simulink model "s_sip_lqr"  (Simulink 7.8)
settings: Solver=ode4  StartTime=0.0  StopTime=10  FixedStep=0.002  RelTol=1e-3  AbsTol=1e-6
values from neighbouring files (symbols this model uses):
  A = [0 0 1 0 ... (first row only)    [SIP_ABCD_eqns.m]
  B = eta_g*Kg*eta_m*Kt/r_mp/Rm*B    [SIP_ABCD_eqns.m]
  C = eye(2,4)    [SIP_ABCD_eqns.m]    (also in d_ip02_sip_lqr.m = eye( 4 ))
  D = zeros(2,1)    [SIP_ABCD_eqns.m]    (also in d_ip02_sip_lqr.m = zeros( 4, 1 ))
  IC_ALPHA0 = IC_ALPHA0 / 180 * pi    (= 0)    [setup_ip02_sip.m]
  wcf = 2 * pi * 10.0    (= 62.8318530718)    [setup_ip02_sip.m]
  zetaf = 0.9    [setup_ip02_sip.m]
undefined symbols (not defined in the file or in its folder): K, VMAX_AMP
libraries: simulink_extras x1, quarc_library x1
settings Model: Creator=MLevis  LastModifiedBy=pmartin  ExtModeTrigDuration=5000  ExtModeArmWhenConnect=off  BufferReuse=off
settings SolverCC: PositivePriorityOrder=on
settings DataIOCC: LimitDataPoints=off
settings OptimizationCC: BooleanDataType=off  OptimizeBlockIOStorage=off  BufferReuse=off  ExpressionFolding=off  FoldNonRolledExpr=off  LocalBlockOutputs=off  InitFltsAndDblsToZero=on
settings DebuggingCC: SaveWithParameterizedLinksMsg=none  SignalResolutionControl=TryResolveAllWithWarning  SolverPrmCheckMsg=none  MultiTaskDSMMsg=warning  MultiTaskCondExecSysMsg=none  FcnCallInpInsideContextMsg=Use local settings  StrictBusMsg=None
settings RTWCC: SystemTargetFile=quarc_windows.tlc  TemplateMakefile=quarc_default_tmf  Description=QUARC Win32 Target  ProcessScript=quarc_windows_make_rtw_hook  IncludeERTFirstTime=on
settings STFCustomTargetCC: TargetFcnLib=ansi_tfl_tmw.mat  TargetPreCompLibLocation=C:\PROGRA~2\QUARC\lib\2011b\windows\release  SystemTargetFile=quarc_windows.tlc
settings GRTTargetCC: TargetFcnLib=ansi_tfl_tmw.mat  TargetPreCompLibLocation=C:\PROGRA~2\QUARC\lib\2011b\windows\release  ParMdlRefBuildCompliant=off  CompOptLevelCompliant=off  ConcurrentExecutionCompliant=off  MatFileLogging=off  ExtMode=on  ExtModeMexFile=quarc_comm

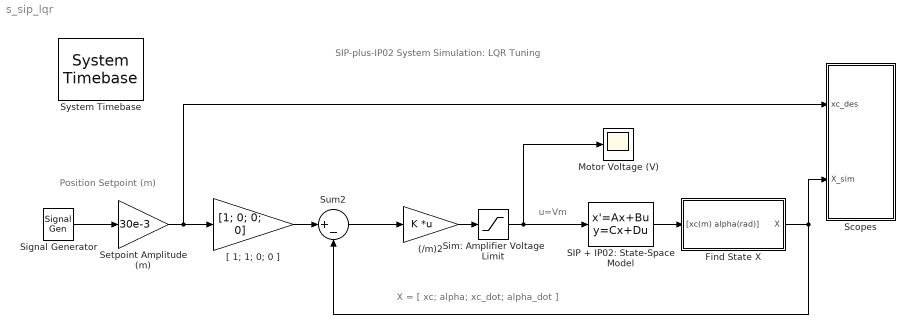
== system s_sip_lqr ==
  note: SIP-plus-IP02 System Simulation:
      | LQR Tuning
  note: Position Setpoint (m)
  note: u=Vm
  note: X = [ xc; alpha; xc_dot; alpha_dot ]
  (/m)2 : Gain  Gain=K  Multiplication=Matrix(K*u)  SaturateOnIntegerOverflow=on  OutDataTypeStr=Inherit: Same as input  ParamDataTypeStr=Inherit: Same as input
  Find State X : Subsystem
  Motor Voltage (V) : Scope
      settings: YMin=-0.6  YMax=0.6  SaveName=data_vm  DataFormat=Array
  SIP + IP02: State-Space Model : StateSpace  A=A  B=B  C=C  D=D  X0=[ 0; IC_ALPHA0; 0; 0 ]
  Scopes : Subsystem
  Setpoint Amplitude (m) : Gain  Gain=30e-3  SaturateOnIntegerOverflow=on  OutDataTypeStr=Inherit: Same as input  ParamDataTypeStr=Inherit: Same as input
  Signal Generator : SignalGenerator  WaveForm=square  Frequency=0.2
  Sim: Amplifier Voltage Limit : Saturate  UpperLimit=VMAX_AMP  LowerLimit=- VMAX_AMP
  Sum2 : Sum  Inputs=|+-  SaturateOnIntegerOverflow=on  InputSameDT=on  OutDataTypeStr=Inherit: Same as first input
  System Timebase : quarc_library/Advanced/Timing/System Timebase  stop_on_overrun=off
  "[ 1; 1; 0; 0 ]" : Gain  Gain=[1; 0; 0; 0]  SaturateOnIntegerOverflow=on  OutDataTypeStr=Inherit: Same as input  ParamDataTypeStr=Inherit: Same as input
  wires:
  Signal Generator/1 -> Setpoint Amplitude (m)/1
  (/m)2/1 -> Sim: Amplifier Voltage Limit/1
  Sum2/1 -> (/m)2/1
  Sim: Amplifier Voltage Limit/1 -> SIP + IP02: State-Space Model/1, Motor Voltage (V)/1
  SIP + IP02: State-Space Model/1 -> Find State X/1("[xc(m) alpha(rad)]")
  Find State X/1(X) -> Sum2/2, Scopes/2(X_sim)
  Setpoint Amplitude (m)/1 -> "[ 1; 1; 0; 0 ]"/1, Scopes/1(xc_des)
  "[ 1; 1; 0; 0 ]"/1 -> Sum2/1

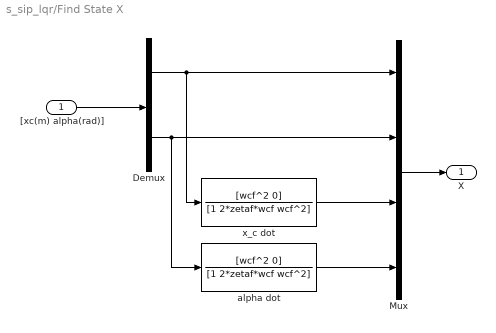
== system s_sip_lqr/Find State X ==
  "[xc(m) alpha(rad)]" : Inport
  Demux : Demux  Outputs=2
  Mux : Mux
  alpha dot : TransferFcn  Numerator=[wcf^2 0]  Denominator=[1 2*zetaf*wcf wcf^2]
  x_c dot : TransferFcn  Numerator=[wcf^2 0]  Denominator=[1 2*zetaf*wcf wcf^2]
  X : Outport
  wires:
  Mux/1 -> X/1
  x_c dot/1 -> Mux/3
  alpha dot/1 -> Mux/4
  "[xc(m) alpha(rad)]"/1 -> Demux/1
  Demux/1 -> Mux/1, x_c dot/1
  Demux/2 -> Mux/2, alpha dot/1

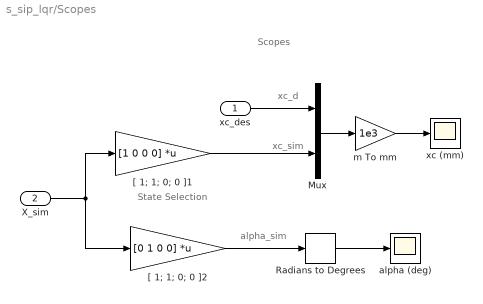
== system s_sip_lqr/Scopes ==
  note: xc_sim
  note: State Selection
  note: alpha_sim
  note: xc_d
  note: Scopes
  xc_des : Inport
  X_sim : Inport  Port=2
  Mux : Mux  Inputs=2
  Radians to Degrees : simulink_extras/Transformations/Radians to Degrees
  "[ 1; 1; 0; 0 ]1" : Gain  Gain=[1 0 0 0]  Multiplication=Matrix(K*u)  SaturateOnIntegerOverflow=on  OutDataTypeStr=Inherit: Same as input  ParamDataTypeStr=Inherit: Same as input
  "[ 1; 1; 0; 0 ]2" : Gain  Gain=[0 1 0 0]  Multiplication=Matrix(K*u)  SaturateOnIntegerOverflow=on  OutDataTypeStr=Inherit: Same as input  ParamDataTypeStr=Inherit: Same as input
  alpha (deg) : Scope
      settings: TickLabels=on  TimeRange=5  YMin=-0.5  YMax=0.5  SaveName=data_alpha  DataFormat=Array
  m To mm : Gain  Gain=1e3  SaturateOnIntegerOverflow=on  OutDataTypeStr=Inherit: Same as input  ParamDataTypeStr=Inherit: Same as input
  xc (mm) : Scope
      settings: TickLabels=on  TimeRange=5  YMin=-25  YMax=25  SaveName=data_xc  DataFormat=Array
  wires:
  Mux/1 -> m To mm/1
  m To mm/1 -> xc (mm)/1
  "[ 1; 1; 0; 0 ]1"/1 -> Mux/2
  xc_des/1 -> Mux/1
  X_sim/1 -> "[ 1; 1; 0; 0 ]1"/1, "[ 1; 1; 0; 0 ]2"/1
  Radians to Degrees/1 -> alpha (deg)/1
  "[ 1; 1; 0; 0 ]2"/1 -> Radians to Degrees/1
